simulink model "afe_abc_inv_psm_2mods"  (R2025a)
settings: Solver=ode1be  StartTime=0.0  StopTime=simlength  FixedStep=tc  MaxStep=tc
undefined symbols (not defined in the file): Ad_fht, Adrso, afe_pwm_phase_shift_mod1, afe_pwm_phase_shift_mod2, Amplitude_U, Amplitude_V, Amplitude_W, Aresd, b, Bresd, Cfht, Cresd, Crso, CTRPIFF_CLIP_RELEASE, dead_time_AFE, dead_time_INV, deepNEGeta, deepNEGxi, deepPOSxi, emf_fb_p, emf_fb_p_ccaller_1, emf_fb_p_ccaller_2, emf_p, emf_p_ccaller_1, emf_p_ccaller_2, enable_two_modules, end_time_LVRT, fPWM_AFE, fPWM_INV, g0_161Hz, g0_500Hz, g1_161Hz, g1_500Hz, i_grid_neg_eta_lim, i_grid_neg_eta_red_lim, i_grid_neg_xi_lim, i_grid_neg_xi_red_lim, i_grid_pos_eta_lim, i_grid_pos_eta_red_lim, ibez, id_lim, ieta_neg_ref_lim, ieta_pos_ref_lim, Igrid_phase_normalization_factor, inv_pwm_phase_shift_mod1, inv_pwm_phase_shift_mod2, iq_lim, ixi_pos_ref_lim, Jm, k_frt_ref, kg, ki_afe, ki_i, ki_rc_neg_grid, ki_rc_pos_grid, ki_vs, ki_w, kp_afe, kp_i, kp_rc_neg_grid ... (+64)
libraries: spsSampleandHoldLib x213, fl_lib x202, nesl_utility x126, simulink x22, cstblocks x18, threephase_inductor_lib x4, single_phase_transformer_lib x3, flexshaft_lib x1, pmsm_uvw_with_harmonics_lib x1
(part 8 of 18)

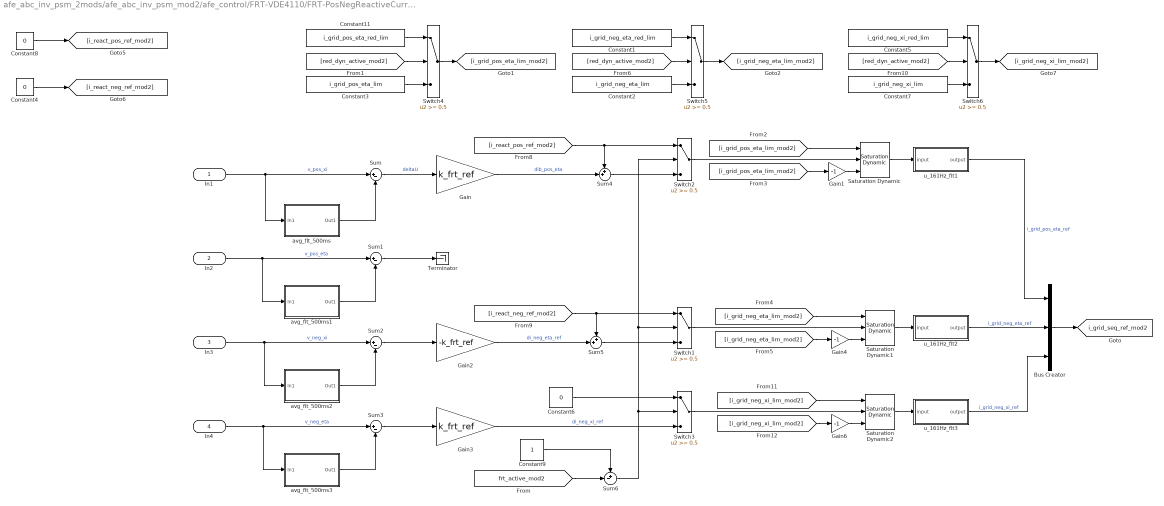
== system afe_abc_inv_psm_2mods/afe_abc_inv_psm_mod2/afe_control/FRT-VDE4110/FRT-PosNegReactiveCurrentReferences ==
  In1 : Inport
  In2 : Inport  Port=2
  In3 : Inport  Port=3
  In4 : Inport  Port=4
  Bus Creator : BusCreator  Inputs=3
  Constant1 : Constant  Value=i_grid_neg_eta_red_lim
  Constant11 : Constant  Value=i_grid_pos_eta_red_lim
  Constant2 : Constant  Value=i_grid_neg_eta_lim
  Constant3 : Constant  Value=i_grid_pos_eta_lim
  Constant4 : Constant  Value=0
  Constant5 : Constant  Value=i_grid_neg_xi_red_lim
  Constant6 : Constant  Value=0
  Constant7 : Constant  Value=i_grid_neg_xi_lim
  Constant8 : Constant  Value=0
  Constant9 : Constant
  Gain : Gain  Gain=k_frt_ref
  Gain1 : Gain  Gain=-1
  Gain2 : Gain  Gain=-k_frt_ref
  Gain3 : Gain  Gain=k_frt_ref
  Gain4 : Gain  Gain=-1
  Gain6 : Gain  Gain=-1
  Saturation Dynamic : simulink/Discontinuities/Saturation Dynamic  OutMin=[]  OutMax=[]  OutDataTypeStr=Inherit: Same as second input  OutDataType=fixdt(1, 16)  OutScaling=2^-10  DoSatur=off
  Saturation Dynamic1 : simulink/Discontinuities/Saturation Dynamic  OutMin=[]  OutMax=[]  OutDataTypeStr=Inherit: Same as second input  OutDataType=fixdt(1, 16)  OutScaling=2^-10  DoSatur=off
  Saturation Dynamic2 : simulink/Discontinuities/Saturation Dynamic  OutMin=[]  OutMax=[]  OutDataTypeStr=Inherit: Same as second input  OutDataType=fixdt(1, 16)  OutScaling=2^-10  DoSatur=off
  Sum{,1..3} (4 alike) : Sum  Inputs=|+-
  Sum4 : Sum  Inputs=++|
  Sum5 : Sum  Inputs=++|
  Sum6 : Sum  Inputs=+-|
  Switch{1..6} (6 alike) : Switch  Threshold=0.5  SaturateOnIntegerOverflow=off  InputSameDT=off
  Terminator : Terminator
  avg_flt_500ms : Subsystem
  avg_flt_500ms1 : Subsystem
  avg_flt_500ms2 : Subsystem
  avg_flt_500ms3 : Subsystem
  u_161Hz_flt1 : Subsystem
  u_161Hz_flt2 : Subsystem
  u_161Hz_flt3 : Subsystem
  tag scope: i_grid_seq_ref_mod2=global
  wires:
  In1/1 -> avg_flt_500ms/1(In1), Sum/1  "v_pos_xi"
  avg_flt_500ms/1(Out1) -> Sum/2
  Sum/1 -> Gain/1  "deltaU"
  Sum1/1 -> Terminator/1
  avg_flt_500ms1/1(Out1) -> Sum1/2
  In2/1 -> avg_flt_500ms1/1(In1), Sum1/1  "v_pos_eta"
  avg_flt_500ms3/1(Out1) -> Sum3/2
  Sum2/1 -> Gain2/1
  In3/1 -> avg_flt_500ms2/1(In1), Sum2/1  "v_neg_xi"
  avg_flt_500ms2/1(Out1) -> Sum2/2
  In4/1 -> avg_flt_500ms3/1(In1), Sum3/1  "v_neg_eta"
  Bus Creator/1 -> [i_grid_seq_ref_mod2]
  Gain/1 -> Sum4/2  "dib_pos_eta"
  [i_react_pos_ref_mod2] -> Switch2/1, Sum4/1
  Sum4/1 -> Switch2/3
  Switch2/1 -> Saturation Dynamic/2
  Saturation Dynamic/1 -> u_161Hz_flt1/1(input)
  Constant6/1 -> Switch3/1
  Gain3/1 -> Switch3/3  "di_neg_xi_ref"
  Sum6/1 -> Switch1/2, Switch2/2, Switch3/2
  Sum3/1 -> Gain3/1
  Gain2/1 -> Sum5/2  "di_neg_eta_ref"
  Sum5/1 -> Switch1/3
  [i_react_neg_ref_mod2] -> Switch1/1, Sum5/1
  Switch4/1 -> [i_grid_pos_eta_lim_mod2]
  [red_dyn_active_mod2] -> Switch4/2
  Constant3/1 -> Switch4/3
  Constant11/1 -> Switch4/1
  [i_grid_pos_eta_lim_mod2] -> Saturation Dynamic/1
  [i_grid_pos_eta_lim_mod2] -> Gain1/1
  Gain1/1 -> Saturation Dynamic/3
  Saturation Dynamic2/1 -> u_161Hz_flt3/1(input)
  Switch3/1 -> Saturation Dynamic2/2
  [i_grid_neg_xi_lim_mod2] -> Saturation Dynamic2/1
  [i_grid_neg_xi_lim_mod2] -> Gain6/1
  Gain4/1 -> Saturation Dynamic1/3
  [i_grid_neg_eta_lim_mod2] -> Gain4/1
  [i_grid_neg_eta_lim_mod2] -> Saturation Dynamic1/1
  Switch1/1 -> Saturation Dynamic1/2
  Saturation Dynamic1/1 -> u_161Hz_flt2/1(input)
  [red_dyn_active_mod2] -> Switch5/2
  Constant2/1 -> Switch5/3
  Constant1/1 -> Switch5/1
  Switch5/1 -> [i_grid_neg_eta_lim_mod2]
  Constant4/1 -> [i_react_neg_ref_mod2]
  Constant8/1 -> [i_react_pos_ref_mod2]
  Constant7/1 -> Switch6/3
  Switch6/1 -> [i_grid_neg_xi_lim_mod2]
  Constant5/1 -> Switch6/1
  [red_dyn_active_mod2] -> Switch6/2
  Gain6/1 -> Saturation Dynamic2/3
  u_161Hz_flt2/1(output) -> Bus Creator/2  "i_grid_neg_eta_ref"
  u_161Hz_flt3/1(output) -> Bus Creator/3  "i_grid_neg_xi_ref"
  u_161Hz_flt1/1(output) -> Bus Creator/1  "i_grid_pos_eta_ref"
  [frt_active_mod2] -> Sum6/2
  Constant9/1 -> Sum6/1

== system afe_abc_inv_psm_2mods/afe_abc_inv_psm_mod2/afe_control/current_ctrl/Inner Loop Current Control ==
  In1 : Inport
  is_abc : Inport  Port=2
  -1<x<1 : Saturate  UpperLimit=1  LowerLimit=-1
  Add : Sum
  Bus Creator1 : BusCreator  Inputs=2
  Demux1 : Demux  Outputs=3
  MATLAB Function : MATLAB Function  TreatAsAtomicUnit=on
  Mux : Mux  Inputs=3
  Selector : Selector  InputPortWidth=3  IndexOptions=Index vector (dialog)  Indices=[1]  OutputSizes=1
  Selector1 : Selector  InputPortWidth=3  IndexOptions=Index vector (dialog)  Indices=[1]  OutputSizes=1
  Selector2 : Selector  InputPortWidth=3  IndexOptions=Index vector (dialog)  Indices=[2]  OutputSizes=1
  Selector3 : Selector  InputPortWidth=3  IndexOptions=Index vector (dialog)  Indices=[2]  OutputSizes=1
  Selector4 : Selector  InputPortWidth=3  IndexOptions=Index vector (dialog)  Indices=[3]  OutputSizes=1
  Selector5 : Selector  InputPortWidth=3  IndexOptions=Index vector (dialog)  Indices=[3]  OutputSizes=1
  Unit Delay1 : UnitDelay  SampleTime=ts_afe  HasFrameUpgradeWarning=on
  Unit Delay2 : UnitDelay  SampleTime=ts_afe  HasFrameUpgradeWarning=on
  Unit Delay3 : UnitDelay  SampleTime=ts_afe  HasFrameUpgradeWarning=on
  isa_ref/isa : Scope  NumInputPorts=2
      settings: SampleTime=ts_afe  ActiveDisplayYMinimum=-1.42299  ActiveDisplayYMaximum=1.07212
  isb_ref/isb : Scope  NumInputPorts=2
      settings: SampleTime=ts_afe  ActiveDisplayYMinimum=-1.02549  ActiveDisplayYMaximum=2.17852  DataLoggingVariableName=ScopeData2
  isc_ref/isc : Scope  NumInputPorts=2
      settings: SampleTime=ts_afe  ActiveDisplayYMinimum=-12.82873  ActiveDisplayYMaximum=11.54837  DataLoggingVariableName=ScopeData3
  rpi-ph-a : Subsystem
  rpi-ph-b : Subsystem
  rpi-ph-c : Subsystem
  uab : Outport  VectorParamsAs1DForOutWhenUnconnected=off
  wires:
  [v_grid_ff_abc_mod2] -> Unit Delay1/1
  -1<x<1/1 -> Demux1/1  "v_abc"
  Bus Creator1/1 -> uab/1
  Unit Delay2/1 -> Bus Creator1/1  "ualpha_afe"
  Demux1/1 -> MATLAB Function/1(a)  "v_a"
  MATLAB Function/2(beta) -> Unit Delay3/1  "u_beta"
  Demux1/2 -> MATLAB Function/2(b)  "v_b"
  Unit Delay3/1 -> Bus Creator1/2  "ubeta_afe"
  MATLAB Function/1(alpha) -> Unit Delay2/1  "u_alpha"
  Demux1/3 -> MATLAB Function/3(c)  "v_c"
  Mux/1 -> Add/1  "v_abc"
  rpi-ph-c/1(Out1) -> Mux/3  "v_c"
  rpi-ph-b/1(Out1) -> Mux/2  "v_b"
  rpi-ph-a/1(Out1) -> Mux/1  "v_a"
  Selector5/1 -> rpi-ph-c/2(In2), isc_ref/isc/2  "isc"
  Selector4/1 -> rpi-ph-c/1(In1), isc_ref/isc/1  "isc_ref"
  Selector3/1 -> rpi-ph-b/2(In2), isb_ref/isb/2  "isb"
  Selector2/1 -> rpi-ph-b/1(In1), isb_ref/isb/1  "isb_ref"
  Selector1/1 -> rpi-ph-a/2(In2), isa_ref/isa/2  "isa"
  Selector/1 -> rpi-ph-a/1(In1), isa_ref/isa/1  "isa_ref"
  Add/1 -> -1<x<1/1  "v_abc"
  is_abc/1 -> Selector1/1, Selector3/1, Selector5/1  "i_abc"
  In1/1 -> Selector/1, Selector2/1, Selector4/1  "i_abc_ref"

== system afe_abc_inv_psm_2mods/afe_abc_inv_psm_mod2/afe_control/current_ctrl/current_transformation ==
  is_a_pu : Inport
  is_b_pu : Inport  Port=2
  is_c_pu : Inport  Port=3
  Bus Creator : BusCreator  Inputs=3
  alphabeta2xieta : MATLAB Function  TreatAsAtomicUnit=on  SystemSampleTime=ts_afe
  uvw2alphabeta : MATLAB Function  TreatAsAtomicUnit=on  SystemSampleTime=ts_afe
  tag scope: i_eta_pu_mod2=global, i_xi_pu_mod2=global, is_abc_pu_mod2=global
  wires:
  Bus Creator/1 -> [is_abc_pu_mod2]
  is_a_pu/1 -> uvw2alphabeta/1(u), Bus Creator/1
  [gamma_grid_pll_mod2] -> alphabeta2xieta/3(gamma)
  uvw2alphabeta/1(alpha) -> alphabeta2xieta/1(alpha)  "ialpha_pu"
  uvw2alphabeta/2(beta) -> alphabeta2xieta/2(beta)  "ibeta_pu"
  is_b_pu/1 -> uvw2alphabeta/2(v), Bus Creator/2
  alphabeta2xieta/1(xi) -> [i_xi_pu_mod2]  "ixi_pu"
  alphabeta2xieta/2(eta) -> [i_eta_pu_mod2]  "ieta_pu"
  is_c_pu/1 -> uvw2alphabeta/3(w), Bus Creator/3

== system afe_abc_inv_psm_2mods/afe_abc_inv_psm_mod2/afe_control/current_ctrl/sample_hold_normalization ==
  is_a : Inport
  is_b : Inport  Port=2
  is_c : Inport  Port=3
  Gain : Gain  Gain=1/Igrid_phase_normalization_factor
  Gain1 : Gain  Gain=1/Igrid_phase_normalization_factor
  Gain2 : Gain  Gain=1/Igrid_phase_normalization_factor
  Quantizer : Quantizer  QuantizationInterval=adc_quantization
  Quantizer1 : Quantizer  QuantizationInterval=adc_quantization
  Quantizer2 : Quantizer  QuantizationInterval=adc_quantization
  Subsystem1 : Subsystem
      mask Display: disp('S/H afe mod 2');
  Subsystem2 : Subsystem
      mask Display: disp('S/H afe mod 2');
  Subsystem5 : Subsystem
      mask Display: disp('S/H afe mod 2');
  Unit Delay : UnitDelay  SampleTime=ts_afe  HasFrameUpgradeWarning=on
  Unit Delay1 : UnitDelay  SampleTime=ts_afe  HasFrameUpgradeWarning=on
  Unit Delay2 : UnitDelay  SampleTime=ts_afe  HasFrameUpgradeWarning=on
  is_a_pu : Outport
  is_b_pu : Outport  Port=2
  is_c_pu : Outport  Port=3
  wires:
  Subsystem5/1(Out) -> Unit Delay2/1
  Subsystem2/1(Out) -> Unit Delay1/1
  Subsystem1/1(Out) -> Unit Delay/1
  Quantizer2/1 -> Subsystem5/1(In)
  Quantizer1/1 -> Subsystem2/1(In)
  Unit Delay2/1 -> is_c_pu/1
  Unit Delay1/1 -> is_b_pu/1
  Unit Delay/1 -> is_a_pu/1
  is_b/1 -> Gain1/1
  is_c/1 -> Gain2/1
  Quantizer/1 -> Subsystem1/1(In)
  is_a/1 -> Gain/1
  Gain/1 -> Quantizer/1
  Gain1/1 -> Quantizer1/1
  Gain2/1 -> Quantizer2/1

== system afe_abc_inv_psm_2mods/afe_abc_inv_psm_mod2/afe_control/current_ctrl/xieta2abc ==
  pos_xi : Inport
  pos_eta : Inport  Port=2
  neg_xi : Inport  Port=3
  neg_eta : Inport  Port=4
  gamma : Inport  Port=5
  MATLAB Function2 : MATLAB Function  TreatAsAtomicUnit=on
  Mux : Mux  Inputs=3
  Negative Sequence : MATLAB Function  TreatAsAtomicUnit=on
  Positive Sequence : MATLAB Function  TreatAsAtomicUnit=on
  Sum : Sum  Inputs=|++
  Sum1 : Sum  Inputs=|++
  i_abc : Outport
  wires:
  Mux/1 -> i_abc/1  "i_abc"
  pos_eta/1 -> Positive Sequence/2(eta)
  pos_xi/1 -> Positive Sequence/1(xi)
  neg_xi/1 -> Negative Sequence/1(xi)
  Sum1/1 -> MATLAB Function2/2(beta)
  MATLAB Function2/2(b) -> Mux/2  "i_b"
  Negative Sequence/2(beta) -> Sum1/2
  Positive Sequence/1(alpha) -> Sum/1
  Negative Sequence/1(alpha) -> Sum/2
  MATLAB Function2/3(c) -> Mux/3  "i_c"
  gamma/1 -> Positive Sequence/3(gamma), Negative Sequence/3(gamma)
  Sum/1 -> MATLAB Function2/1(alpha)
  Positive Sequence/2(beta) -> Sum1/1
  MATLAB Function2/1(a) -> Mux/1  "i_a"
  neg_eta/1 -> Negative Sequence/2(eta)

== system afe_abc_inv_psm_2mods/afe_abc_inv_psm_mod2/afe_control/current_sequence_avg/average_filter_ccaller ==
  i_grid_pos_xi : Inport
  i_grid_pos_eta : Inport  Port=2
  i_grid_neg_xi : Inport  Port=3
  i_grid_neg_eta : Inport  Port=4
  Moving Average Filter1 : Subsystem
  Moving Average Filter2 : Subsystem
  Moving Average Filter3 : Subsystem
  Moving Average Filter5 : Subsystem
  i_grid_pos_xi_avg : Outport
  i_grid_pos_eta_avg : Outport  Port=2
  i_grid_neg_xi_avg : Outport  Port=3
  i_grid_neg_eta_avg : Outport  Port=4
  wires:
  Moving Average Filter5/1(xi) -> i_grid_pos_xi_avg/1
  i_grid_neg_eta/1 -> Moving Average Filter3/1(In2)
  i_grid_pos_xi/1 -> Moving Average Filter5/1(In2)
  Moving Average Filter2/1(xi) -> i_grid_neg_xi_avg/1
  i_grid_neg_xi/1 -> Moving Average Filter2/1(In2)
  Moving Average Filter3/1(xi) -> i_grid_neg_eta_avg/1
  i_grid_pos_eta/1 -> Moving Average Filter1/1(In2)
  [omega_grid_pll_mod2] -> Moving Average Filter1/2(In3), Moving Average Filter3/2(In3), Moving Average Filter2/2(In3), Moving Average Filter5/2(In3)
  Moving Average Filter1/1(xi) -> i_grid_pos_eta_avg/1

== system afe_abc_inv_psm_2mods/afe_abc_inv_psm_mod2/afe_control/current_sequence_avg/average_filter_simulink ==
  i_grid_pos_xi : Inport
  i_grid_pos_eta : Inport  Port=2
  i_grid_neg_xi : Inport  Port=3
  i_grid_neg_eta : Inport  Port=4
  moving_avarage_1 : Subsystem
  moving_avarage_2 : Subsystem
  moving_avarage_3 : Subsystem
  moving_avarage_4 : Subsystem
  i_grid_pos_xi_avg : Outport
  i_grid_pos_eta_avg : Outport  Port=2
  i_grid_neg_xi_avg : Outport  Port=3
  i_grid_neg_eta_avg : Outport  Port=4
  wires:
  i_grid_pos_eta/1 -> moving_avarage_2/1(in)
  i_grid_neg_eta/1 -> moving_avarage_4/1(in)
  i_grid_pos_xi/1 -> moving_avarage_1/1(in)
  i_grid_neg_xi/1 -> moving_avarage_3/1(in)
  moving_avarage_4/1(out) -> i_grid_neg_eta_avg/1
  moving_avarage_1/1(out) -> i_grid_pos_xi_avg/1
  moving_avarage_2/1(out) -> i_grid_pos_eta_avg/1
  moving_avarage_3/1(out) -> i_grid_neg_xi_avg/1

== system afe_abc_inv_psm_2mods/afe_abc_inv_psm_mod2/afe_control/grid_current_sampling_and_alpha_beta_transformation/sample_hold_normalization ==
  ig_a : Inport
  ig_b : Inport  Port=2
  ig_c : Inport  Port=3
  Gain1 : Gain  Gain=1/Igrid_phase_normalization_factor
  Gain2 : Gain  Gain=1/Igrid_phase_normalization_factor
  Gain3 : Gain  Gain=1/Igrid_phase_normalization_factor
  Gain4 : Gain  Gain=-1
  Gain5 : Gain  Gain=-1
  Gain6 : Gain  Gain=-1
  Quantizer1 : Quantizer  QuantizationInterval=adc_quantization
  Quantizer2 : Quantizer  QuantizationInterval=adc_quantization
  Quantizer4 : Quantizer  QuantizationInterval=adc_quantization
  Subsystem1 : Subsystem
      mask Display: disp('S/H afe mod 2');
  Subsystem2 : Subsystem
      mask Display: disp('S/H afe mod 2');
  Subsystem5 : Subsystem
      mask Display: disp('S/H afe mod 2');
  Unit Delay : UnitDelay  SampleTime=ts_afe  HasFrameUpgradeWarning=on
  Unit Delay1 : UnitDelay  SampleTime=ts_afe  HasFrameUpgradeWarning=on
  Unit Delay2 : UnitDelay  SampleTime=ts_afe  HasFrameUpgradeWarning=on
  ig_a_pu : Outport
  ig_b_pu : Outport  Port=2
  ig_c_pu : Outport  Port=3
  wires:
  Unit Delay2/1 -> Gain4/1
  Unit Delay1/1 -> Gain5/1
  Unit Delay/1 -> Gain6/1
  ig_c/1 -> Gain2/1
  ig_b/1 -> Gain1/1
  ig_a/1 -> Gain3/1
  Gain2/1 -> Quantizer2/1
  Gain1/1 -> Quantizer1/1
  Gain3/1 -> Quantizer4/1
  Quantizer2/1 -> Subsystem5/1(In)
  Quantizer1/1 -> Subsystem2/1(In)
  Quantizer4/1 -> Subsystem1/1(In)
  Subsystem5/1(Out) -> Unit Delay2/1
  Subsystem1/1(Out) -> Unit Delay/1
  Subsystem2/1(Out) -> Unit Delay1/1
  Gain6/1 -> ig_a_pu/1
  Gain5/1 -> ig_b_pu/1
  Gain4/1 -> ig_c_pu/1

== system afe_abc_inv_psm_2mods/afe_abc_inv_psm_mod2/afe_control/grid_voltage_phase_lock_loops/DDSRF-PLL ==
  pll_stageA : Subsystem
  pll_stageB : Subsystem
  grid_phase_out : Outport
  wires:
  pll_stageA/1(u_grid_pos_xi) -> pll_stageB/1(u_grid_pos_xi)  "u_grid_pos_xi"
  pll_stageA/2(u_grid_pos_eta) -> pll_stageB/2(u_grid_pos_eta)  "u_grid_pos_eta"
  pll_stageB/1(wt_grid) -> grid_phase_out/1, pll_stageA/1(gamma_grid)

== system afe_abc_inv_psm_2mods/afe_abc_inv_psm_mod2/afe_control/grid_voltage_phase_lock_loops/DQ-PLL ==
  pll_stageA : Subsystem
  pll_stageB : Subsystem
  grid_phase_out : Outport
  wires:
  pll_stageA/1(u_grid_pos_xi) -> pll_stageB/1(u_grid_pos_xi)  "u_grid_pos_xi"
  pll_stageB/1(gamma_grid_pll) -> grid_phase_out/1, pll_stageA/1(gamma_grid)
  pll_stageA/2(u_grid_pos_eta) -> pll_stageB/2(u_grid_pos_eta)  "u_grid_pos_eta"

== system afe_abc_inv_psm_2mods/afe_abc_inv_psm_mod2/afe_control/grid_voltage_sampling_and_alpha_beta_transformation/sample_hold_normalization ==
  vg_a : Inport
  vg_b : Inport  Port=2
  vg_c : Inport  Port=3
  Gain : Gain  Gain=1/Vgrid_phase_normalization_factor
  Gain1 : Gain  Gain=1/Vgrid_phase_normalization_factor
  Gain2 : Gain  Gain=1/Vgrid_phase_normalization_factor
  Quantizer1 : Quantizer  QuantizationInterval=adc_quantization
  Quantizer2 : Quantizer  QuantizationInterval=adc_quantization
  Quantizer4 : Quantizer  QuantizationInterval=adc_quantization
  Subsystem1 : Subsystem
      mask Display: disp('S/H afe mod 2');
  Subsystem2 : Subsystem
      mask Display: disp('S/H afe mod 2');
  Subsystem6 : Subsystem
      mask Display: disp('S/H afe mod 2');
  Unit Delay : UnitDelay  SampleTime=ts_afe  HasFrameUpgradeWarning=on
  Unit Delay1 : UnitDelay  SampleTime=ts_afe  HasFrameUpgradeWarning=on
  Unit Delay2 : UnitDelay  SampleTime=ts_afe  HasFrameUpgradeWarning=on
  vg_a_pu : Outport
  vg_b_pu : Outport  Port=2
  vg_c_pu : Outport  Port=3
  wires:
  Quantizer2/1 -> Subsystem2/1(In)
  Quantizer1/1 -> Subsystem1/1(In)
  Quantizer4/1 -> Subsystem6/1(In)
  Gain/1 -> Quantizer4/1
  Gain1/1 -> Quantizer1/1
  Gain2/1 -> Quantizer2/1
  Subsystem2/1(Out) -> Unit Delay2/1
  Subsystem1/1(Out) -> Unit Delay1/1
  Subsystem6/1(Out) -> Unit Delay/1
  vg_c/1 -> Gain2/1
  vg_b/1 -> Gain1/1
  Unit Delay2/1 -> vg_c_pu/1
  Unit Delay1/1 -> vg_b_pu/1
  Unit Delay/1 -> vg_a_pu/1
  vg_a/1 -> Gain/1

== system afe_abc_inv_psm_2mods/afe_abc_inv_psm_mod2/afe_control/sequences_current_control/Negative-Seq. eta-Control ==
  ff : Inport
  e : Inport  Port=2
  1/Ti : Gain  Gain=kp_rc_neg_grid  SaturateOnIntegerOverflow=on  OutDataTypeStr=Inherit: Same as input  ParamDataTypeStr=Inherit: Same as input
  Saturation : Saturate  UpperLimit=ieta_neg_ref_lim  LowerLimit=-ieta_neg_ref_lim
  Sum : Sum  Inputs=|++
  Sum2 : Sum  Inputs=+++  SaturateOnIntegerOverflow=on
  Sum3 : Sum  Inputs=-+  SaturateOnIntegerOverflow=on
  Unit Delay4 : UnitDelay  SampleTime=ts_afe  HasFrameUpgradeWarning=on
  kp : Gain  Gain=ki_rc_neg_grid*ts_afe  SaturateOnIntegerOverflow=on  OutDataTypeStr=Inherit: Same as input  ParamDataTypeStr=Inherit: Same as input
  u : Outport  VectorParamsAs1DForOutWhenUnconnected=off
  wires:
  ff/1 -> Sum/2
  e/1 -> kp/1, 1/Ti/1  "e"
  Sum/1 -> u/1
  Saturation/1 -> Sum3/2, Sum/1
  1/Ti/1 -> Sum3/1, Sum2/1
  Sum2/1 -> Saturation/1
  kp/1 -> Sum2/2
  Sum3/1 -> Unit Delay4/1
  Unit Delay4/1 -> Sum2/3

== system afe_abc_inv_psm_2mods/afe_abc_inv_psm_mod2/afe_control/sequences_current_control/Negative-Seq. xi-Control ==
  ff : Inport
  e : Inport  Port=2
  1/Ti : Gain  Gain=kp_rc_neg_grid  SaturateOnIntegerOverflow=on  OutDataTypeStr=Inherit: Same as input  ParamDataTypeStr=Inherit: Same as input
  Saturation : Saturate  UpperLimit=ieta_pos_ref_lim  LowerLimit=-ieta_pos_ref_lim
  Sum : Sum  Inputs=|++
  Sum2 : Sum  Inputs=+++  SaturateOnIntegerOverflow=on
  Sum3 : Sum  Inputs=-+  SaturateOnIntegerOverflow=on
  Unit Delay4 : UnitDelay  SampleTime=ts_afe  HasFrameUpgradeWarning=on
  kp : Gain  Gain=ki_rc_neg_grid*ts_afe  SaturateOnIntegerOverflow=on  OutDataTypeStr=Inherit: Same as input  ParamDataTypeStr=Inherit: Same as input
  u : Outport  VectorParamsAs1DForOutWhenUnconnected=off
  wires:
  ff/1 -> Sum/2
  e/1 -> kp/1, 1/Ti/1  "e"
  Sum/1 -> u/1
  Saturation/1 -> Sum3/2, Sum/1
  1/Ti/1 -> Sum3/1, Sum2/1
  Sum2/1 -> Saturation/1
  kp/1 -> Sum2/2
  Sum3/1 -> Unit Delay4/1
  Unit Delay4/1 -> Sum2/3

== system afe_abc_inv_psm_2mods/afe_abc_inv_psm_mod2/afe_control/sequences_current_control/Positive-Seq. eta-Control ==
  ff : Inport
  e : Inport  Port=2
  1/Ti : Gain  Gain=kp_rc_pos_grid  SaturateOnIntegerOverflow=on  OutDataTypeStr=Inherit: Same as input  ParamDataTypeStr=Inherit: Same as input
  Saturation : Saturate  UpperLimit=ieta_pos_ref_lim  LowerLimit=-ieta_pos_ref_lim
  Sum : Sum  Inputs=|++
  Sum2 : Sum  Inputs=+++  SaturateOnIntegerOverflow=on
  Sum3 : Sum  Inputs=-+  SaturateOnIntegerOverflow=on
  Unit Delay4 : UnitDelay  SampleTime=ts_afe  HasFrameUpgradeWarning=on
  kp : Gain  Gain=ki_rc_pos_grid*ts_afe  SaturateOnIntegerOverflow=on  OutDataTypeStr=Inherit: Same as input  ParamDataTypeStr=Inherit: Same as input
  u : Outport  VectorParamsAs1DForOutWhenUnconnected=off
  wires:
  ff/1 -> Sum/2
  e/1 -> kp/1, 1/Ti/1  "e"
  Sum/1 -> u/1
  Saturation/1 -> Sum3/2, Sum/1
  1/Ti/1 -> Sum3/1, Sum2/1
  Sum2/1 -> Saturation/1
  kp/1 -> Sum2/2
  Sum3/1 -> Unit Delay4/1
  Unit Delay4/1 -> Sum2/3

== system afe_abc_inv_psm_2mods/afe_abc_inv_psm_mod2/afe_control/voltage_sequence_avg/average_filter_ccaller ==
  v_grid_pos_xi : Inport
  v_grid_pos_eta : Inport  Port=2
  v_grid_neg_xi : Inport  Port=3
  v_grid_neg_eta : Inport  Port=4
  Moving Average Filter1 : Subsystem
  Moving Average Filter2 : Subsystem
  Moving Average Filter3 : Subsystem
  Moving Average Filter4 : Subsystem
  v_grid_pos_xi_avg : Outport
  v_grid_pos_eta_avg : Outport  Port=2
  v_grid_neg_xi_avg : Outport  Port=3
  v_grid_neg_eta_avg : Outport  Port=4
  wires:
  v_grid_pos_eta/1 -> Moving Average Filter2/1(In2)
  Moving Average Filter1/1(xi) -> v_grid_pos_xi_avg/1
  Moving Average Filter4/1(xi) -> v_grid_neg_eta_avg/1
  Moving Average Filter3/1(xi) -> v_grid_neg_xi_avg/1
  v_grid_neg_eta/1 -> Moving Average Filter4/1(In2)
  v_grid_neg_xi/1 -> Moving Average Filter3/1(In2)
  v_grid_pos_xi/1 -> Moving Average Filter1/1(In2)
  [omega_grid_pll_mod1] -> Moving Average Filter2/2(In3), Moving Average Filter4/2(In3), Moving Average Filter3/2(In3), Moving Average Filter1/2(In3)
  Moving Average Filter2/1(xi) -> v_grid_pos_eta_avg/1

== system afe_abc_inv_psm_2mods/afe_abc_inv_psm_mod2/afe_control/voltage_sequence_avg/average_filter_simulink ==
  v_grid_pos_xi : Inport
  v_grid_pos_eta : Inport  Port=2
  v_grid_neg_xi : Inport  Port=3
  v_grid_neg_eta : Inport  Port=4
  moving_avarage_1 : Subsystem
  moving_avarage_2 : Subsystem
  moving_avarage_3 : Subsystem
  moving_avarage_4 : Subsystem
  v_grid_pos_xi_avg : Outport
  v_grid_pos_eta_avg : Outport  Port=2
  v_grid_neg_xi_avg : Outport  Port=3
  v_grid_neg_eta_avg : Outport  Port=4
  wires:
  v_grid_pos_eta/1 -> moving_avarage_2/1(in)
  v_grid_neg_eta/1 -> moving_avarage_4/1(in)
  v_grid_pos_xi/1 -> moving_avarage_1/1(in)
  v_grid_neg_xi/1 -> moving_avarage_3/1(in)
  moving_avarage_4/1(out) -> v_grid_neg_eta_avg/1
  moving_avarage_1/1(out) -> v_grid_pos_xi_avg/1
  moving_avarage_2/1(out) -> v_grid_pos_eta_avg/1
  moving_avarage_3/1(out) -> v_grid_neg_xi_avg/1

== system afe_abc_inv_psm_2mods/afe_abc_inv_psm_mod2/inverter/inverter/sv_pwm ==
  ab : Inport
  enable : Inport  Port=2
  Bus Selector : BusSelector  OutputSignals=da,db,dc
  Bus Selector1 : BusSelector  OutputSignals=ua,ub
  C Caller : CCaller  FunctionName=sv_pwm_process_simulink  PortSpecificationStruct="%)30     .    N @   8    (     @         %    \"     4    !     0         %  0 \"0    $    _    07)G3F%M90  4&]R=$YA;64 4V-O<&4     26YD97@     5'EP90      4VEZ90      27-';&]B86P   X    P    !@    @    $          4    (     0    ,    !         !   P!O=70 #@   #     &    \"     0         !0    @    !     P    $         $  # &]U=  .    .     8    (    !          %    \"     $    &     0         0   ...(+2630 chars)"  SampleTime=ts_inv
  Constant : Constant  Value=ts_inv
  Constant1 : Constant  Value=inv_pwm_phase_shift_mod2
  Data Type Conversion1 : DataTypeConversion  OutDataTypeStr=double  SaturateOnIntegerOverflow=off  RndMeth=Floor
  Data Type Conversion15 : DataTypeConversion  OutDataTypeStr=single  SaturateOnIntegerOverflow=off  RndMeth=Floor
  Data Type Conversion16 : DataTypeConversion  OutDataTypeStr=single  SaturateOnIntegerOverflow=off  RndMeth=Floor
  Data Type Conversion17 : DataTypeConversion  OutDataTypeStr=uint32  SaturateOnIntegerOverflow=off  RndMeth=Floor
  Data Type Conversion18 : DataTypeConversion  OutDataTypeStr=single  SaturateOnIntegerOverflow=off  RndMeth=Floor
  Data Type Conversion2 : DataTypeConversion  OutDataTypeStr=double  SaturateOnIntegerOverflow=off  RndMeth=Floor
  Data Type Conversion3 : DataTypeConversion  OutDataTypeStr=double  SaturateOnIntegerOverflow=off  RndMeth=Floor
  Gain : Gain  Gain=sqrt(3)/2
  Gain1 : Gain  Gain=sqrt(3)/2
  Subsystem1 : Subsystem
      mask Display: disp('S/H inv mod 1');
  Subsystem2 : Subsystem
      mask Display: disp('S/H inv mod 1');
  Subsystem3 : Subsystem
      mask Display: disp('S/H inv mod 1');
  Subsystem4 : Subsystem
      mask Display: disp('S/H inv mod 1');
  modulator1 : Subsystem
  sv2pwm_inv : Scope  NumInputPorts=2
      settings: ActiveDisplayYMinimum=0.14692  ActiveDisplayYMaximum=0.85308  DataLoggingVariableName=ScopeData2
  firing_gates : Outport
  wires:
  Bus Selector/3 -> Data Type Conversion3/1  "<dc>"
  Bus Selector/2 -> Data Type Conversion2/1  "<db>"
  Bus Selector/1 -> Data Type Conversion1/1  "<da>"
  Gain1/1 -> Data Type Conversion15/1
  Gain/1 -> Data Type Conversion18/1
  Subsystem4/1(Out) -> C Caller/4
  Subsystem3/1(Out) -> C Caller/3
  Subsystem2/1(Out) -> C Caller/2
  Subsystem1/1(Out) -> C Caller/1
  Bus Selector1/2 -> Gain1/1  "<ub>"
  Bus Selector1/1 -> Gain/1  "<ua>"
  ab/1 -> Bus Selector1/1, sv2pwm_inv/2
  modulator1/1(cmd_gates) -> firing_gates/1
  Data Type Conversion3/1 -> modulator1/3(w)  "dw"
  C Caller/1 -> sv2pwm_inv/1, Bus Selector/1  "out"
  Data Type Conversion17/1 -> Subsystem4/1(In)
  Data Type Conversion15/1 -> Subsystem2/1(In)
  Data Type Conversion2/1 -> modulator1/2(v)  "dv"
  enable/1 -> Data Type Conversion17/1
  Constant/1 -> Data Type Conversion16/1
  Data Type Conversion16/1 -> Subsystem3/1(In)
  Data Type Conversion18/1 -> Subsystem1/1(In)
  Data Type Conversion1/1 -> modulator1/1(u)  "du"
  Constant1/1 -> modulator1/4(phase)

== system afe_abc_inv_psm_2mods/afe_abc_inv_psm_mod2/inverter/inverter/switch_1 ==
  Diode : fl_lib/Electrical/Electrical Elements/Diode  Vf=Vgamma V  Ron=Ron Ohm  Goff=1e-8 1/Ohm  i_specify=off  i_priority=None  i=0 A  i_nominal_specify=off  i_nominal_value=1  i_nominal_unit=A  v_specify=off  v_priority=None  v=0 V  v_nominal_specify=off  v_nominal_value=1  v_nominal_unit=V
  Switch : fl_lib/Electrical/Electrical Elements/Switch  R_closed=Ron Ohm  G_open=1e-8 1/Ohm  Threshold=7.5  i_specify=off  i_priority=None  i=0 A  i_nominal_specify=off  i_nominal_value=1  i_nominal_unit=A  v_specify=off  v_priority=None  v=0 V  v_nominal_specify=off  v_nominal_value=1  v_nominal_unit=V
  G : PMIOPort  Side=Left
  C : PMIOPort  Port=2  Side=Left
  E : PMIOPort  Port=3  Side=Right
  connections:
  Diode/LConn1 -- E/RConn1 -- Switch/LConn1
  Switch/RConn1 -- G/RConn1
  Diode/RConn1 -- C/RConn1 -- Switch/RConn2

== system afe_abc_inv_psm_2mods/afe_abc_inv_psm_mod2/inverter/inverter/switch_2 ==
  Diode : fl_lib/Electrical/Electrical Elements/Diode  Vf=Vgamma V  Ron=Ron Ohm  Goff=1e-8 1/Ohm  i_specify=off  i_priority=None  i=0 A  i_nominal_specify=off  i_nominal_value=1  i_nominal_unit=A  v_specify=off  v_priority=None  v=0 V  v_nominal_specify=off  v_nominal_value=1  v_nominal_unit=V
  Switch : fl_lib/Electrical/Electrical Elements/Switch  R_closed=Ron Ohm  G_open=1e-8 1/Ohm  Threshold=7.5  i_specify=off  i_priority=None  i=0 A  i_nominal_specify=off  i_nominal_value=1  i_nominal_unit=A  v_specify=off  v_priority=None  v=0 V  v_nominal_specify=off  v_nominal_value=1  v_nominal_unit=V
  G : PMIOPort  Side=Left
  C : PMIOPort  Port=2  Side=Left
  E : PMIOPort  Port=3  Side=Right
  connections:
  Switch/RConn2 -- C/RConn1 -- Diode/RConn1
  Switch/RConn1 -- G/RConn1
  Switch/LConn1 -- E/RConn1 -- Diode/LConn1

== system afe_abc_inv_psm_2mods/afe_abc_inv_psm_mod2/inverter/inverter/switch_3 ==
  Diode : fl_lib/Electrical/Electrical Elements/Diode  Vf=Vgamma V  Ron=Ron Ohm  Goff=1e-8 1/Ohm  i_specify=off  i_priority=None  i=0 A  i_nominal_specify=off  i_nominal_value=1  i_nominal_unit=A  v_specify=off  v_priority=None  v=0 V  v_nominal_specify=off  v_nominal_value=1  v_nominal_unit=V
  Switch : fl_lib/Electrical/Electrical Elements/Switch  R_closed=Ron Ohm  G_open=1e-8 1/Ohm  Threshold=7.5  i_specify=off  i_priority=None  i=0 A  i_nominal_specify=off  i_nominal_value=1  i_nominal_unit=A  v_specify=off  v_priority=None  v=0 V  v_nominal_specify=off  v_nominal_value=1  v_nominal_unit=V
  G : PMIOPort  Side=Left
  C : PMIOPort  Port=2  Side=Left
  E : PMIOPort  Port=3  Side=Right
  connections:
  Switch/RConn2 -- C/RConn1 -- Diode/RConn1
  Switch/RConn1 -- G/RConn1
  Switch/LConn1 -- E/RConn1 -- Diode/LConn1

== system afe_abc_inv_psm_2mods/afe_abc_inv_psm_mod2/inverter/inverter/switch_4 ==
  Diode : fl_lib/Electrical/Electrical Elements/Diode  Vf=Vgamma V  Ron=Ron Ohm  Goff=1e-8 1/Ohm  i_specify=off  i_priority=None  i=0 A  i_nominal_specify=off  i_nominal_value=1  i_nominal_unit=A  v_specify=off  v_priority=None  v=0 V  v_nominal_specify=off  v_nominal_value=1  v_nominal_unit=V
  Switch : fl_lib/Electrical/Electrical Elements/Switch  R_closed=Ron Ohm  G_open=1e-8 1/Ohm  Threshold=7.5  i_specify=off  i_priority=None  i=0 A  i_nominal_specify=off  i_nominal_value=1  i_nominal_unit=A  v_specify=off  v_priority=None  v=0 V  v_nominal_specify=off  v_nominal_value=1  v_nominal_unit=V
  G : PMIOPort  Side=Left
  C : PMIOPort  Port=2  Side=Left
  E : PMIOPort  Port=3  Side=Right
  connections:
  Diode/LConn1 -- E/RConn1 -- Switch/LConn1
  Switch/RConn1 -- G/RConn1
  Diode/RConn1 -- C/RConn1 -- Switch/RConn2

== system afe_abc_inv_psm_2mods/afe_abc_inv_psm_mod2/inverter/inverter/switch_5 ==
  Diode : fl_lib/Electrical/Electrical Elements/Diode  Vf=Vgamma V  Ron=Ron Ohm  Goff=1e-8 1/Ohm  i_specify=off  i_priority=None  i=0 A  i_nominal_specify=off  i_nominal_value=1  i_nominal_unit=A  v_specify=off  v_priority=None  v=0 V  v_nominal_specify=off  v_nominal_value=1  v_nominal_unit=V
  Switch : fl_lib/Electrical/Electrical Elements/Switch  R_closed=Ron Ohm  G_open=1e-8 1/Ohm  Threshold=7.5  i_specify=off  i_priority=None  i=0 A  i_nominal_specify=off  i_nominal_value=1  i_nominal_unit=A  v_specify=off  v_priority=None  v=0 V  v_nominal_specify=off  v_nominal_value=1  v_nominal_unit=V
  G : PMIOPort  Side=Left
  C : PMIOPort  Port=2  Side=Left
  E : PMIOPort  Port=3  Side=Right
  connections:
  Switch/RConn2 -- C/RConn1 -- Diode/RConn1
  Switch/RConn1 -- G/RConn1
  Switch/LConn1 -- E/RConn1 -- Diode/LConn1

== system afe_abc_inv_psm_2mods/afe_abc_inv_psm_mod2/inverter/inverter/switch_6 ==
  Diode : fl_lib/Electrical/Electrical Elements/Diode  Vf=Vgamma V  Ron=Ron Ohm  Goff=1e-8 1/Ohm  i_specify=off  i_priority=None  i=0 A  i_nominal_specify=off  i_nominal_value=1  i_nominal_unit=A  v_specify=off  v_priority=None  v=0 V  v_nominal_specify=off  v_nominal_value=1  v_nominal_unit=V
  Switch : fl_lib/Electrical/Electrical Elements/Switch  R_closed=Ron Ohm  G_open=1e-8 1/Ohm  Threshold=7.5  i_specify=off  i_priority=None  i=0 A  i_nominal_specify=off  i_nominal_value=1  i_nominal_unit=A  v_specify=off  v_priority=None  v=0 V  v_nominal_specify=off  v_nominal_value=1  v_nominal_unit=V
  G : PMIOPort  Side=Left
  C : PMIOPort  Port=2  Side=Left
  E : PMIOPort  Port=3  Side=Right
  connections:
  Diode/LConn1 -- E/RConn1 -- Switch/LConn1
  Switch/RConn1 -- G/RConn1
  Diode/RConn1 -- C/RConn1 -- Switch/RConn2

== system afe_abc_inv_psm_2mods/afe_abc_inv_psm_mod2/inverter_control/current_ctrl/bemf_observer ==
  ialpha_pu : Inport
  ibeta_pu : Inport  Port=2
  ualpha_pu : Inport  Port=3
  ubeta_pu : Inport  Port=4
  BEMF Observer simulink/Ccaller module 2 : Scope  NumInputPorts=2
      settings: SampleTime=tc  ActiveDisplayYMinimum=-0.27432  ActiveDisplayYMaximum=0.92036
  Mux : Mux  Inputs=3
  Mux1 : Mux  Inputs=3
  Variant Source : VariantSource  VariantControls={use_observer_from_simulink_module_2 == 1, use_observer_from_ccaller_module_2 == 1}
  Variant Source1 : VariantSource  VariantControls={use_observer_from_simulink_module_2 == 1, use_observer_from_ccaller_module_2 == 1}
  bemf_observer : Subsystem
  bemf_observer_ccaller : Subsystem
  phase_fault : Subsystem  Commented=on
  tag scope: omega_hat_pu_mod2=global, theta_hat_mod2=global
  wires:
  phase_fault/2(theta_hat_encoder) -> Mux1/3
  phase_fault/1(omega_pu_encoder) -> Mux/3
  Variant Source/1 -> [omega_hat_pu_mod2]
  Variant Source1/1 -> [theta_hat_mod2]
  bemf_observer/2(theta_hat) -> Mux1/1, Variant Source1/1  "theta_hat"
  bemf_observer_ccaller/1(omega_pu) -> Variant Source/2, Mux/2  "omega_pu_code"
  bemf_observer_ccaller/2(theta_hat) -> Variant Source1/2, Mux1/2  "theta_hat_code"
  bemf_observer/1(omega_pu) -> Variant Source/1, Mux/1  "omega_pu"
  ubeta_pu/1 -> bemf_observer_ccaller/4(ubeta_pu), bemf_observer/4(ubeta_pu)
  ualpha_pu/1 -> bemf_observer_ccaller/3(ualpha_pu), bemf_observer/3(ualpha_pu)
  Mux1/1 -> BEMF Observer simulink/Ccaller module 2/2
  Mux/1 -> BEMF Observer simulink/Ccaller module 2/1
  ibeta_pu/1 -> bemf_observer_ccaller/2(ibeta_pu), bemf_observer/2(ibeta_pu)
  ialpha_pu/1 -> bemf_observer_ccaller/1(ialpha_pu), bemf_observer/1(ialpha_pu)

== system afe_abc_inv_psm_2mods/afe_abc_inv_psm_mod2/inverter_control/current_ctrl/current_ctrl ==
  iq_ref : Inport
  MTPA : Subsystem
  Sqrt : Sqrt
  Square : Math  Operator=square
  Square1 : Math  Operator=square
  Sum : Sum  Inputs=|++
  To Workspace1 : ToWorkspace  VariableName=id_pu_sim_mod2  SampleTime=ts_inv
      settings: MaxDataPoints=Ns_inv
  To Workspace2 : ToWorkspace  VariableName=iq_pu_sim_mod2  SampleTime=ts_inv
      settings: MaxDataPoints=Ns_inv
  To Workspace3 : ToWorkspace  VariableName=id_ref_pu_sim_mod2  SampleTime=ts_inv
      settings: MaxDataPoints=Ns_inv
  To Workspace4 : ToWorkspace  VariableName=iq_ref_pu_sim_mod2  SampleTime=ts_inv
      settings: MaxDataPoints=Ns_inv
  To Workspace5 : ToWorkspace  VariableName=ud_pu_sim_mod2  SampleTime=ts_inv
      settings: MaxDataPoints=Ns_inv
  To Workspace6 : ToWorkspace  VariableName=uq_pu_sim_mod2  SampleTime=ts_inv
      settings: MaxDataPoints=Ns_inv
  To Workspace7 : ToWorkspace  VariableName=u_mot_pu_sim_mod2  SampleTime=ts_inv
      settings: MaxDataPoints=Ns_inv
  dq_pi_with_vector_antiwindup : Subsystem
  id_ref : Subsystem
      settings: PortSchema="{\"entries\":[{\"content\":{\"sides\":[{\"content\":{},\"type\":\"ConnectorPlacement.EquallySpacedRectSide\",\"uuid\":\"42af5d69-f0eb-42c6-9e03-28c1d0757323\"},{\"content\":{\"connectorIds\":[\"Out1\"],\"side\":\"RIGHT\"},\"type\":\"ConnectorPlacement.EquallySpacedRectSide\",\"uuid\":\"dd68a9f9-d15f-4e57-9d9e-130889a7b90c\"},{\"content\":{\"connectorIds\":[\"In1\"],\"side\":\"TOP\"},\"type\":\"ConnectorPlacement.EquallySpacedRectSide\",\"uuid\":\"68c797a2-8439-4b8d-8368-b7485adf0676\"}]},\"type\":\"ConnectorPlacement.EquallySpacedConnector\",\"uuid\":\"693c5f1c-0580-4626-8f13-b27865dfb3ac\"}],\"packageUris\":[\"http://schema.mathworks.com/mf0/Connector/R2020b\"],\"version\":\"1.0\"}"
  idref/id mod2 : Scope  NumInputPorts=2
      settings: SampleTime=tc  ActiveDisplayYMinimum=-0.56823  ActiveDisplayYMaximum=0.06368
  iqref/iq mod2 : Scope  NumInputPorts=2
      settings: SampleTime=tc  ActiveDisplayYMinimum=-0.28565  ActiveDisplayYMaximum=0.01726  DataLoggingVariableName=ScopeData2
  ud : Outport
  uq : Outport  Port=2
  tag scope: id_pu_ref_mod2=global, iq_pu_ref_mod2=global, u_mot_pu_sim_mod2=global, ud_pu_sim_mod2=global, uq_pu_sim_mod2=global
  wires:
  id_ref/1(id_ref) -> idref/id mod2/1, dq_pi_with_vector_antiwindup/1(id_ref), To Workspace3/1
  Sqrt/1 -> To Workspace7/1, [u_mot_pu_sim_mod2]
  Square1/1 -> Sum/2
  Sum/1 -> Sqrt/1
  Square/1 -> Sum/1
  dq_pi_with_vector_antiwindup/2(ctrl_q_u) -> uq/1, [uq_pu_sim_mod2], To Workspace6/1, Square/1
  dq_pi_with_vector_antiwindup/1(ctrl_d_u) -> ud/1, To Workspace5/1, [ud_pu_sim_mod2], Square1/1
  iq_ref/1 -> [iq_pu_ref_mod2], dq_pi_with_vector_antiwindup/3(iq_ref), iqref/iq mod2/1, To Workspace4/1, MTPA/1(iq_ref)  "iq_ref"
  MTPA/1(Id_ref_mtpa) -> [id_pu_ref_mod2], id_ref/1(id_mtpa)  "id_ref"
  [id_pu_mod2] -> dq_pi_with_vector_antiwindup/2(id), idref/id mod2/2, To Workspace1/1  "id"
  [iq_pu_mod2] -> dq_pi_with_vector_antiwindup/4(iq), iqref/iq mod2/2, To Workspace2/1  "iq"

== system afe_abc_inv_psm_2mods/afe_abc_inv_psm_mod2/inverter_control/current_ctrl/current_transformation ==
  u : Inport
  v : Inport  Port=2
  w : Inport  Port=3
  To Workspace2 : ToWorkspace  VariableName=ialpha_pu_sim_mod2  SampleTime=ts_inv
      settings: MaxDataPoints=Ns_inv
  To Workspace3 : ToWorkspace  VariableName=ibeta_pu_sim_mod2  SampleTime=ts_inv
      settings: MaxDataPoints=Ns_inv
  alphabeta2dq : MATLAB Function  TreatAsAtomicUnit=on  SystemSampleTime=ts_inv
  uvw2alphabeta : MATLAB Function  TreatAsAtomicUnit=on  SystemSampleTime=ts_inv
  tag scope: ialpha_pu_mod2=global, ibeta_pu_mod2=global, id_pu_mod2=global, iq_pu_mod2=global
  wires:
  u/1 -> uvw2alphabeta/1(u)
  [theta_hat_mod2] -> alphabeta2dq/3(gamma)
  uvw2alphabeta/1(alpha) -> alphabeta2dq/1(alpha), [ialpha_pu_mod2], To Workspace2/1  "ialpha_pu"
  uvw2alphabeta/2(beta) -> alphabeta2dq/2(beta), [ibeta_pu_mod2], To Workspace3/1  "ibeta_pu"
  v/1 -> uvw2alphabeta/2(v)
  alphabeta2dq/1(d) -> [id_pu_mod2]  "id_pu"
  alphabeta2dq/2(q) -> [iq_pu_mod2]  "iq_pu"
  w/1 -> uvw2alphabeta/3(w)

== system afe_abc_inv_psm_2mods/afe_abc_inv_psm_mod2/inverter_control/current_ctrl/sample_hold_normalization ==
  iu : Inport
  iv : Inport  Port=2
  iw : Inport  Port=3
  Gain : Gain  Gain=1/ibez
  Gain1 : Gain  Gain=1/ibez
  Gain2 : Gain  Gain=1/ibez
  Gain3 : Gain  Gain=-1
  Gain4 : Gain  Gain=-1
  Gain5 : Gain  Gain=-1
  Quantizer1 : Quantizer  QuantizationInterval=adc_quantization
  Quantizer2 : Quantizer  QuantizationInterval=adc_quantization
  Quantizer4 : Quantizer  QuantizationInterval=adc_quantization
  Subsystem1 : Subsystem
      mask Display: disp('S/H inv mod 2');
  Subsystem2 : Subsystem
      mask Display: disp('S/H inv mod 2');
  Subsystem5 : Subsystem
      mask Display: disp('S/H inv mod 2');
  Unit Delay : UnitDelay  SampleTime=ts_inv  HasFrameUpgradeWarning=on
  Unit Delay1 : UnitDelay  SampleTime=ts_inv  HasFrameUpgradeWarning=on
  Unit Delay4 : UnitDelay  SampleTime=ts_inv  HasFrameUpgradeWarning=on
  iu_pu : Outport
  iv_pu : Outport  Port=2
  iw_pu : Outport  Port=3
  wires:
  Gain5/1 -> iw_pu/1
  Gain4/1 -> iv_pu/1
  Gain3/1 -> iu_pu/1
  Quantizer2/1 -> Subsystem1/1(In)
  Quantizer1/1 -> Subsystem2/1(In)
  Quantizer4/1 -> Subsystem5/1(In)
  Gain2/1 -> Quantizer2/1
  Gain1/1 -> Quantizer1/1
  Gain/1 -> Quantizer4/1
  Subsystem1/1(Out) -> Unit Delay4/1
  Subsystem2/1(Out) -> Unit Delay1/1
  Subsystem5/1(Out) -> Unit Delay/1
  Unit Delay/1 -> Gain3/1
  Unit Delay1/1 -> Gain4/1
  Unit Delay4/1 -> Gain5/1
  iu/1 -> Gain/1
  iw/1 -> Gain2/1
  iv/1 -> Gain1/1

== system afe_abc_inv_psm_2mods/grid/grid_emulator/grid_emulator/phase_gen ==
  Constant4 : Constant  Value=omega_grid_emulator_nom
  Integrator : Integrator
  To Workspace7 : ToWorkspace  VariableName=gamma_grid_emulator_sim  SampleTime=ts_afe
      settings: MaxDataPoints=Ns_afe
  bounder1 : MATLAB Function  TreatAsAtomicUnit=on  SystemSampleTime=ts_afe
  grid_emu_phase : Outport  VectorParamsAs1DForOutWhenUnconnected=off
  tag scope: gamma_grid_emulator=global
  wires:
  bounder1/1(y) -> [gamma_grid_emulator], To Workspace7/1, grid_emu_phase/1  "grid_emu_phase"
  Constant4/1 -> Integrator/1
  Integrator/1 -> bounder1/1(u)

== system afe_abc_inv_psm_2mods/grid/grid_emulator/grid_emulator/voltage_reference ==
  grid_emu_phase : Inport
  Vxi_p : Inport  Port=2
  Vxi_n : Inport  Port=3
  Veta_n : Inport  Port=4
  Constant2 : Constant  Value=0
  Sum1 : Sum  Inputs=|++
  Sum4 : Sum  Inputs=|++
  Variant Source : VariantSource  VariantControls={enable_frt_2 == 1, enable_frt_1 == 1}
  Variant Source1 : VariantSource  VariantControls={enable_frt_2 == 1, enable_frt_1 == 1}
  Variant Source2 : VariantSource  VariantControls={enable_frt_2 == 1, enable_frt_1 == 1}
  alphabeta2abc : MATLAB Function  TreatAsAtomicUnit=on  SystemSampleTime=ts_afe
  voltage_dource_with_frt : Subsystem
  xieta2alphabeta_neg : MATLAB Function  TreatAsAtomicUnit=on  SystemSampleTime=ts_afe
  xieta2alphabeta_pos : MATLAB Function  TreatAsAtomicUnit=on  SystemSampleTime=ts_afe
  V1_ref : Outport  VectorParamsAs1DForOutWhenUnconnected=off
  V2_ref : Outport  Port=2  VectorParamsAs1DForOutWhenUnconnected=off
  V3_ref : Outport  Port=3  VectorParamsAs1DForOutWhenUnconnected=off
  wires:
  xieta2alphabeta_pos/1(alpha) -> Sum1/1
  Sum1/1 -> alphabeta2abc/1(alpha)
  xieta2alphabeta_pos/2(beta) -> Sum4/1
  Sum4/1 -> alphabeta2abc/2(beta)
  xieta2alphabeta_neg/1(alpha) -> Sum1/2
  xieta2alphabeta_neg/2(beta) -> Sum4/2
  grid_emu_phase/1 -> voltage_dource_with_frt/1(gamma), xieta2alphabeta_neg/3(gamma), xieta2alphabeta_pos/3(gamma)
  Vxi_p/1 -> xieta2alphabeta_pos/1(xi)
  Constant2/1 -> xieta2alphabeta_pos/2(eta)
  Vxi_n/1 -> xieta2alphabeta_neg/1(xi)
  Veta_n/1 -> xieta2alphabeta_neg/2(eta)
  Variant Source/1 -> V1_ref/1
  alphabeta2abc/1(a) -> [V1_ref_xieta]
  alphabeta2abc/2(b) -> [V2_ref_xieta]
  alphabeta2abc/3(c) -> [V3_ref_xieta]
  voltage_dource_with_frt/3(vn_eta) -> [V3_ref_abc]
  voltage_dource_with_frt/2(vn_xi) -> [V2_ref_abc]
  voltage_dource_with_frt/1(vp_xi) -> [V1_ref_abc]
  [V1_ref_xieta] -> Variant Source/1
  [V1_ref_abc] -> Variant Source/2
  Variant Source1/1 -> V2_ref/1
  [V2_ref_xieta] -> Variant Source1/1
  [V2_ref_abc] -> Variant Source1/2
  Variant Source2/1 -> V3_ref/1
  [V3_ref_abc] -> Variant Source2/2
  [V3_ref_xieta] -> Variant Source2/1

== system afe_abc_inv_psm_2mods/grid/grid_emulator/grid_emulator/voltage_source ==
  Add10 : Sum  Inputs=+-+
  Add11 : Sum  Inputs=+-+
  Add12 : Sum  Inputs=+-+
  Constant : Constant  Value=vp_xi_pu
  Constant1 : Constant  Value=vn_xi_pu
  Constant2 : Constant  Value=vn_eta_pu
  Gain1 : Gain  Gain=V_phase_normalization_factor
  Gain2 : Gain  Gain=ugrid_factor
  Gain3 : Gain  Gain=ugrid_factor
  Gain4 : Gain  Gain=ugrid_factor
  Gain7 : Gain  Gain=V_phase_normalization_factor
  Gain8 : Gain  Gain=V_phase_normalization_factor
  LTI System1 : cstblocks/LTI System  sys=LVRT_flt_ss_c  IC=[0]  PadeOrder=0
  LTI System2 : cstblocks/LTI System  sys=LVRT_flt_ss_c  IC=[0]  PadeOrder=0
  LTI System3 : cstblocks/LTI System  sys=LVRT_flt_ss_c  IC=[]  PadeOrder=0
  LTI System4 : cstblocks/LTI System  sys=LVRT_flt_ss_c  IC=[]  PadeOrder=0
  LTI System5 : cstblocks/LTI System  sys=LVRT_flt_ss_c  IC=[]  PadeOrder=0
  LTI System6 : cstblocks/LTI System  sys=LVRT_flt_ss_c  IC=[0]  PadeOrder=0
  Rate Limiter{1..9} (9 alike) : RateLimiter  RisingSlewLimit=Vemu_ref_norm/t_ramp  FallingSlewLimit=-Vemu_ref_norm/t_ramp  SampleTimeMode=inherited
  Step10 : Step  Time=end_time_LVRT  After=vp_xi_pu*deepPOSxi  SampleTime=0
  Step11 : Step  Time=0  After=vn_eta_pu  SampleTime=0
  Step12 : Step  Time=start_time_LVRT  After=deepNEGeta  SampleTime=0
  Step13 : Step  Time=end_time_LVRT  After=deepNEGeta  SampleTime=0
  Step5 : Step  Time=0  After=vn_xi_pu  SampleTime=0
  Step6 : Step  Time=start_time_LVRT  After=deepNEGxi  SampleTime=0
  Step7 : Step  Time=end_time_LVRT  After=deepNEGxi  SampleTime=0
  Step8 : Step  Time=0  After=vp_xi_pu  SampleTime=0
  Step9 : Step  Time=start_time_LVRT  After=vp_xi_pu*deepPOSxi  SampleTime=0
  vp_xi : Outport  VectorParamsAs1DForOutWhenUnconnected=off
  vn_xi : Outport  Port=2  VectorParamsAs1DForOutWhenUnconnected=off
  vn_eta : Outport  Port=3  VectorParamsAs1DForOutWhenUnconnected=off
  wires:
  LTI System3/1 -> Gain7/1
  LTI System4/1 -> Gain8/1
  Gain7/1 -> Gain2/1
  Gain8/1 -> Gain3/1
  Gain1/1 -> Gain4/1
  LTI System5/1 -> Gain1/1
  Gain2/1 -> vp_xi/1
  Gain3/1 -> vn_xi/1
  Gain4/1 -> vn_eta/1
  LTI System6/1 -> LTI System5/1
  LTI System1/1 -> LTI System4/1
  LTI System2/1 -> LTI System3/1
  Rate Limiter2/1 -> Add11/3
  Add12/1 -> LTI System6/1
  Step7/1 -> Rate Limiter6/1
  Step6/1 -> Rate Limiter5/1
  Rate Limiter5/1 -> Add10/2
  Step5/1 -> Rate Limiter4/1
  Add11/1 -> LTI System2/1
  Rate Limiter7/1 -> Add12/1
  Step8/1 -> Rate Limiter3/1
  Step12/1 -> Rate Limiter8/1
  Step11/1 -> Rate Limiter7/1
  Rate Limiter1/1 -> Add11/2
  Step9/1 -> Rate Limiter1/1
  Rate Limiter3/1 -> Add11/1
  Rate Limiter8/1 -> Add12/2
  Rate Limiter9/1 -> Add12/3
  Rate Limiter4/1 -> Add10/1
  Rate Limiter6/1 -> Add10/3
  Step10/1 -> Rate Limiter2/1
  Add10/1 -> LTI System1/1
  Step13/1 -> Rate Limiter9/1

== system afe_abc_inv_psm_2mods/afe_abc_inv_psm_mod1/afe/sv_pwm/modulator1/PWM generator 1 ==
  m_index : Inport
  phase : Inport  Port=2
  Constant : Constant  Value=dead_time*f
  Constant1 : Constant  Value=polarity
  Constant2 : Constant  Value=1/f
  Constant4 : Constant
  Data Type Conversion1 : DataTypeConversion
  Data Type Conversion2 : DataTypeConversion
  Gain4 : Gain  Gain=1/2
  Gain5 : Gain  Gain=1/(pi/2)
  Hit Crossing : HitCross  ShowOutputPort=off
  Hit Crossing1 : HitCross  ShowOutputPort=off
  MATLAB Function : MATLAB Function  TreatAsAtomicUnit=on
  Relational Operator1 : RelationalOperator  Operator=<=  InputSameDT=off
  Relational Operator2 : RelationalOperator  Operator=<=  InputSameDT=off
  Relay : Relay  OnOutputValue=pos_cmd_gate  OffOutputValue=neg_cmd_gate
  Relay1 : Relay  OnOutputValue=pos_cmd_gate  OffOutputValue=neg_cmd_gate
  Saturation1 : Saturate  UpperLimit=m_up  LowerLimit=m_low
  Sum : Sum  Inputs=|++  SaturateOnIntegerOverflow=on
  Sum1 : Sum  Inputs=-+|  SaturateOnIntegerOverflow=on
  Sum3 : Sum  Inputs=|++
  Switch : Switch  Criteria=u2 > Threshold  SaturateOnIntegerOverflow=off  InputSameDT=off
  Switch1 : Switch  Criteria=u2 > Threshold  SaturateOnIntegerOverflow=off  InputSameDT=off
  m1 : Outport
  m2 : Outport  Port=2
  wires:
  Relational Operator1/1 -> Data Type Conversion1/1
  m_index/1 -> Saturation1/1
  Relational Operator2/1 -> Data Type Conversion2/1
  Data Type Conversion2/1 -> Switch/1, Switch1/3, Hit Crossing1/1
  Constant/1 -> Sum/2, Sum1/1
  Saturation1/1 -> Sum/1, Sum1/2
  Sum/1 -> Relational Operator1/1
  Sum1/1 -> Relational Operator2/2
  Gain4/1 -> Relational Operator2/1, Relational Operator1/2
  Data Type Conversion1/1 -> Hit Crossing/1, Switch/3, Switch1/1
  Switch/1 -> Relay/1
  Constant2/1 -> MATLAB Function/3(period)
  phase/1 -> MATLAB Function/2(phase)
  MATLAB Function/1(y) -> Gain5/1
  Gain5/1 -> Sum3/1
  Sum3/1 -> Gain4/1
  Constant4/1 -> Sum3/2
  Relay/1 -> m2/1
  Constant1/1 -> Switch1/2, Switch/2
  Switch1/1 -> Relay1/1
  Relay1/1 -> m1/1
  [time_afe_module_1] -> MATLAB Function/1(t)
